simulink model "Acquisition_from_autosave"  (R2017a)
settings: Solver=VariableStepAuto  StartTime=0.0  StopTime=0.5  RelTol=1e-3
undefined symbols (not defined in the file): magnitude, Radix
libraries: simulink x34, commfilt2 x30, dspswit3 x12, dspmtrx3 x12, dspxfrm3 x3, simulink_extras x2, dspbuff3 x1
(part 3 of 4)

== system Acquisition_from_autosave/Tracking Loop/Tracking Loops/Tracking Loop3/Code Filter/Coeffiecients ==
  BW : Inport
  Zeta : Inport  Port=2
  ts : Inport  Port=3
  Constant1 : Constant  Value=2
  Divide1 : Product  Inputs=**/
  Math Function : Math  Operator=square  SaturateOnIntegerOverflow=on
  Math Function1 : Math  Operator=reciprocal  SaturateOnIntegerOverflow=on
  Wn : Subsystem
  "calc1 " : Subsystem
  calc2 : Product  Inputs=/*
  C1 : Outport
  C2 : Outport  Port=2
  wires:
  BW/1 -> Wn/1(BW)
  Zeta/1 -> Divide1/2, Wn/2(Zeta)
  Math Function/1 -> Math Function1/1
  Constant1/1 -> "calc1 "/1(2), Divide1/1
  Math Function1/1 -> "calc1 "/3(t1), calc2/1
  "calc1 "/1(Out1) -> C1/1
  calc2/1 -> C2/1
  Divide1/1 -> "calc1 "/2(t2)
  Wn/1(Wn) -> Divide1/3, Math Function/1
  ts/1 -> "calc1 "/4(ts), calc2/2

== system Acquisition_from_autosave/Tracking Loop/Tracking Loops/Tracking Loop3/PRN Generator /CA_Code  ==
  In1 : Inport
  CA_Code : MATLAB Function  TreatAsAtomicUnit=on  SystemSampleTime=0.001
  Constant1 : Constant  Value=32
  RT : RateTransition  OutPortSampleTime=0.001
  Reshape : Reshape  OutputDimensionality=Column vector (2-D)
  Out1 : Outport
  wires:
  In1/1 -> RT/1
  CA_Code/1(g) -> Reshape/1
  Constant1/1 -> CA_Code/2(fs)
  Reshape/1 -> Out1/1
  RT/1 -> CA_Code/1(sv)

== system Acquisition_from_autosave/Tracking Loop/Tracking Loops/Tracking Loop3/PRN Generator /NRZ ==
  In1 : Inport
  Constant5 : Constant  Value=2  SampleTime=-1
  Constant6 : Constant  Value=-1
  Product4 : Product
  Sum4 : Sum  Inputs=|++
  Out1 : Outport
  wires:
  Constant6/1 -> Sum4/1
  Sum4/1 -> Out1/1
  Product4/1 -> Sum4/2
  In1/1 -> Product4/2
  Constant5/1 -> Product4/1

== system Acquisition_from_autosave/Tracking Loop/Tracking Loops/Tracking Loop4/Carrier Filter/Filter Parameters ==
  BW : Constant  Value=25
  Constant : Constant  Value=8
  Constant1 : Constant  Value=4
  Constant2 : Constant
  Constant3 : Constant  Value=2
  Damping : Constant  Value=0.707
  Divide : Product  Inputs=*/
  Gain 1 : Product  Inputs=***/
  Gain 2 : Product  Inputs=**/
  K : Constant
  Product : Product  Inputs=3
  Product1 : Product  Inputs=3
  Sum : Sum  Inputs=|++
  K1 : Outport
  K2 : Outport  Port=2
  wires:
  Damping/1 -> Gain 1/3, Product1/2, Product1/1, Product/3
  K/1 -> Gain 2/3, Gain 1/4
  BW/1 -> Product/2
  Constant/1 -> Product/1
  Product/1 -> Divide/1
  Constant1/1 -> Product1/3
  Constant2/1 -> Sum/1
  Product1/1 -> Sum/2
  Sum/1 -> Divide/2
  Divide/1 -> Gain 2/2, Gain 2/1, Gain 1/1
  Constant3/1 -> Gain 1/2
  Gain 1/1 -> K1/1
  Gain 2/1 -> K2/1

== system Acquisition_from_autosave/Tracking Loop/Tracking Loops/Tracking Loop4/Carrier Filter/Subsystem ==
  BW : Constant  Value=30
  C1 : Subsystem
  C2 : Subsystem
  Constant1 : Constant  Value=8
  Constant2 : Constant  Value=4
  Constant4 : Constant
  Damping : Constant  Value=0.707
  K : Constant  Value=4
  T : Constant  Value=0.001
  Wn : Subsystem
  "K2 " : Outport
  K1 : Outport  Port=2
  wires:
  C1/1(Out1) -> K1/1
  Constant1/1 -> C1/1(In1), Wn/1(In1)
  BW/1 -> Wn/2(In2)
  Damping/1 -> C1/2(In2), C1/3(In3), Wn/3(In3), C2/3(In3), C2/2(In2)
  Constant2/1 -> C2/5(In5), C1/7(In7), C2/6(In6), C2/7(In7), C1/8(In8), Wn/4(In4)
  Constant4/1 -> Wn/5(In5)
  T/1 -> C1/4(In4), C1/5(In5), C1/6(In6), C2/4(In4)
  Wn/1(Out1) -> C1/10(In10), C2/8(In8), C1/9(In9)
  C2/1(Out1) -> "K2 "/1
  K/1 -> C1/11(In11), C2/1(In1)

== system Acquisition_from_autosave/Tracking Loop/Tracking Loops/Tracking Loop4/Code Filter/Coeffiecients ==
  BW : Inport
  Zeta : Inport  Port=2
  ts : Inport  Port=3
  Constant1 : Constant  Value=2
  Divide1 : Product  Inputs=**/
  Math Function : Math  Operator=square  SaturateOnIntegerOverflow=on
  Math Function1 : Math  Operator=reciprocal  SaturateOnIntegerOverflow=on
  Wn : Subsystem
  "calc1 " : Subsystem
  calc2 : Product  Inputs=/*
  C1 : Outport
  C2 : Outport  Port=2
  wires:
  BW/1 -> Wn/1(BW)
  Zeta/1 -> Divide1/2, Wn/2(Zeta)
  Math Function/1 -> Math Function1/1
  Constant1/1 -> "calc1 "/1(2), Divide1/1
  Math Function1/1 -> "calc1 "/3(t1), calc2/1
  "calc1 "/1(Out1) -> C1/1
  calc2/1 -> C2/1
  Divide1/1 -> "calc1 "/2(t2)
  Wn/1(Wn) -> Divide1/3, Math Function/1
  ts/1 -> "calc1 "/4(ts), calc2/2

== system Acquisition_from_autosave/Tracking Loop/Tracking Loops/Tracking Loop4/PRN Generator /CA_Code  ==
  In1 : Inport
  CA_Code : MATLAB Function  TreatAsAtomicUnit=on  SystemSampleTime=0.001
  Constant1 : Constant  Value=32
  RT : RateTransition  OutPortSampleTime=0.001
  Reshape : Reshape  OutputDimensionality=Column vector (2-D)
  Out1 : Outport
  wires:
  In1/1 -> RT/1
  CA_Code/1(g) -> Reshape/1
  Constant1/1 -> CA_Code/2(fs)
  Reshape/1 -> Out1/1
  RT/1 -> CA_Code/1(sv)

== system Acquisition_from_autosave/Tracking Loop/Tracking Loops/Tracking Loop4/PRN Generator /NRZ ==
  In1 : Inport
  Constant5 : Constant  Value=2  SampleTime=-1
  Constant6 : Constant  Value=-1
  Product4 : Product
  Sum4 : Sum  Inputs=|++
  Out1 : Outport
  wires:
  Constant6/1 -> Sum4/1
  Sum4/1 -> Out1/1
  Product4/1 -> Sum4/2
  In1/1 -> Product4/2
  Constant5/1 -> Product4/1

== system Acquisition_from_autosave/Tracking Loop/Tracking Loops/Tracking Loop5/Carrier Filter/Filter Parameters ==
  BW : Constant  Value=25
  Constant : Constant  Value=8
  Constant1 : Constant  Value=4
  Constant2 : Constant
  Constant3 : Constant  Value=2
  Damping : Constant  Value=0.707
  Divide : Product  Inputs=*/
  Gain 1 : Product  Inputs=***/
  Gain 2 : Product  Inputs=**/
  K : Constant
  Product : Product  Inputs=3
  Product1 : Product  Inputs=3
  Sum : Sum  Inputs=|++
  K1 : Outport
  K2 : Outport  Port=2
  wires:
  Damping/1 -> Gain 1/3, Product1/2, Product1/1, Product/3
  K/1 -> Gain 2/3, Gain 1/4
  BW/1 -> Product/2
  Constant/1 -> Product/1
  Product/1 -> Divide/1
  Constant1/1 -> Product1/3
  Constant2/1 -> Sum/1
  Product1/1 -> Sum/2
  Sum/1 -> Divide/2
  Divide/1 -> Gain 2/2, Gain 2/1, Gain 1/1
  Constant3/1 -> Gain 1/2
  Gain 1/1 -> K1/1
  Gain 2/1 -> K2/1

== system Acquisition_from_autosave/Tracking Loop/Tracking Loops/Tracking Loop5/Carrier Filter/Subsystem ==
  BW : Constant  Value=30
  C1 : Subsystem
  C2 : Subsystem
  Constant1 : Constant  Value=8
  Constant2 : Constant  Value=4
  Constant4 : Constant
  Damping : Constant  Value=0.707
  K : Constant  Value=4
  T : Constant  Value=0.001
  Wn : Subsystem
  "K2 " : Outport
  K1 : Outport  Port=2
  wires:
  C1/1(Out1) -> K1/1
  Constant1/1 -> C1/1(In1), Wn/1(In1)
  BW/1 -> Wn/2(In2)
  Damping/1 -> C1/2(In2), C1/3(In3), Wn/3(In3), C2/3(In3), C2/2(In2)
  Constant2/1 -> C2/5(In5), C1/7(In7), C2/6(In6), C2/7(In7), C1/8(In8), Wn/4(In4)
  Constant4/1 -> Wn/5(In5)
  T/1 -> C1/4(In4), C1/5(In5), C1/6(In6), C2/4(In4)
  Wn/1(Out1) -> C1/10(In10), C2/8(In8), C1/9(In9)
  C2/1(Out1) -> "K2 "/1
  K/1 -> C1/11(In11), C2/1(In1)

== system Acquisition_from_autosave/Tracking Loop/Tracking Loops/Tracking Loop5/Code Filter/Coeffiecients ==
  BW : Inport
  Zeta : Inport  Port=2
  ts : Inport  Port=3
  Constant1 : Constant  Value=2
  Divide1 : Product  Inputs=**/
  Math Function : Math  Operator=square  SaturateOnIntegerOverflow=on
  Math Function1 : Math  Operator=reciprocal  SaturateOnIntegerOverflow=on
  Wn : Subsystem
  "calc1 " : Subsystem
  calc2 : Product  Inputs=/*
  C1 : Outport
  C2 : Outport  Port=2
  wires:
  BW/1 -> Wn/1(BW)
  Zeta/1 -> Divide1/2, Wn/2(Zeta)
  Math Function/1 -> Math Function1/1
  Constant1/1 -> "calc1 "/1(2), Divide1/1
  Math Function1/1 -> "calc1 "/3(t1), calc2/1
  "calc1 "/1(Out1) -> C1/1
  calc2/1 -> C2/1
  Divide1/1 -> "calc1 "/2(t2)
  Wn/1(Wn) -> Divide1/3, Math Function/1
  ts/1 -> "calc1 "/4(ts), calc2/2

== system Acquisition_from_autosave/Tracking Loop/Tracking Loops/Tracking Loop5/PRN Generator /CA_Code  ==
  In1 : Inport
  CA_Code : MATLAB Function  TreatAsAtomicUnit=on  SystemSampleTime=0.001
  Constant1 : Constant  Value=32
  RT : RateTransition  OutPortSampleTime=0.001
  Reshape : Reshape  OutputDimensionality=Column vector (2-D)
  Out1 : Outport
  wires:
  In1/1 -> RT/1
  CA_Code/1(g) -> Reshape/1
  Constant1/1 -> CA_Code/2(fs)
  Reshape/1 -> Out1/1
  RT/1 -> CA_Code/1(sv)

== system Acquisition_from_autosave/Tracking Loop/Tracking Loops/Tracking Loop5/PRN Generator /NRZ ==
  In1 : Inport
  Constant5 : Constant  Value=2  SampleTime=-1
  Constant6 : Constant  Value=-1
  Product4 : Product
  Sum4 : Sum  Inputs=|++
  Out1 : Outport
  wires:
  Constant6/1 -> Sum4/1
  Sum4/1 -> Out1/1
  Product4/1 -> Sum4/2
  In1/1 -> Product4/2
  Constant5/1 -> Product4/1

== system Acquisition_from_autosave/Tracking Loop/Tracking Loops/Tracking Loop1/Carrier Filter/Subsystem/C1 ==
  In1 : Inport
  In2 : Inport  Port=2
  In3 : Inport  Port=3
  In4 : Inport  Port=4
  In5 : Inport  Port=5
  In6 : Inport  Port=6
  In7 : Inport  Port=7
  In8 : Inport  Port=8
  In9 : Inport  Port=9
  In10 : Inport  Port=10
  In11 : Inport  Port=11
  Add1 : Sum  Inputs=+++
  Gain 3 : Product  Inputs=***/
  Gain 4 : Product  Inputs=***
  Math Function3 : Math  Operator=square  SaturateOnIntegerOverflow=on
  Product3 : Product
  Product4 : Product  Inputs=4
  Out1 : Outport
  wires:
  In5/1 -> Product4/4
  In7/1 -> Add1/3
  Gain 3/1 -> Out1/1
  In9/1 -> Product4/3
  In4/1 -> Product3/1
  In8/1 -> Product4/1
  In2/1 -> Gain 4/1
  In11/1 -> Gain 3/1
  In10/1 -> Product3/2, Gain 4/2
  In1/1 -> Gain 3/3
  In6/1 -> Gain 4/3
  In3/1 -> Product4/2
  Add1/1 -> Gain 3/4
  Product4/1 -> Add1/2
  Gain 4/1 -> Gain 3/2
  Math Function3/1 -> Add1/1
  Product3/1 -> Math Function3/1

== system Acquisition_from_autosave/Tracking Loop/Tracking Loops/Tracking Loop1/Carrier Filter/Subsystem/C2 ==
  In1 : Inport
  In2 : Inport  Port=2
  In3 : Inport  Port=3
  In4 : Inport  Port=4
  In5 : Inport  Port=5
  In6 : Inport  Port=6
  In7 : Inport  Port=7
  In8 : Inport  Port=8
  Add : Sum  Inputs=+++
  Gain 1 : Product  Inputs=***/
  Gain 2 : Product  Inputs=***
  Math Function : Math  Operator=square  SaturateOnIntegerOverflow=on
  Math Function1 : Math  Operator=square  SaturateOnIntegerOverflow=on
  Product1 : Product
  Product2 : Product  Inputs=4
  Out1 : Outport
  wires:
  Product1/1 -> Math Function1/1
  Math Function1/1 -> Add/1
  Add/1 -> Gain 1/4
  In2/1 -> Gain 2/1
  In5/1 -> Add/3
  In7/1 -> Product2/1
  In3/1 -> Product2/2
  In1/1 -> Gain 1/3
  In6/1 -> Gain 1/2
  Product2/1 -> Add/2
  Gain 1/1 -> Out1/1
  Math Function/1 -> Gain 1/1
  In8/1 -> Product1/1, Gain 2/2, Product2/3
  In4/1 -> Product1/2, Product2/4, Gain 2/3
  Gain 2/1 -> Math Function/1

== system Acquisition_from_autosave/Tracking Loop/Tracking Loops/Tracking Loop1/Carrier Filter/Subsystem/Wn ==
  In1 : Inport
  In2 : Inport  Port=2
  In3 : Inport  Port=3
  In4 : Inport  Port=4
  In5 : Inport  Port=5
  Add : Sum
  Divide1 : Product  Inputs=***/
  Math Function : Math  Operator=square  SaturateOnIntegerOverflow=on
  Wn1 : Product
  Out1 : Outport
  wires:
  In4/1 -> Wn1/2
  Add/1 -> Divide1/4
  Wn1/1 -> Add/1
  In3/1 -> Divide1/3, Math Function/1
  In2/1 -> Divide1/2
  Math Function/1 -> Wn1/1
  Divide1/1 -> Out1/1
  In1/1 -> Divide1/1
  In5/1 -> Add/2

== system Acquisition_from_autosave/Tracking Loop/Tracking Loops/Tracking Loop1/Filter/Subsystem/C1 ==
  In1 : Inport
  In2 : Inport  Port=2
  In3 : Inport  Port=3
  In4 : Inport  Port=4
  In5 : Inport  Port=5
  In6 : Inport  Port=6
  In7 : Inport  Port=7
  In8 : Inport  Port=8
  In9 : Inport  Port=9
  In10 : Inport  Port=10
  In11 : Inport  Port=11
  Add1 : Sum  Inputs=+++
  Gain 3 : Product  Inputs=***/
  Gain 4 : Product  Inputs=***
  Math Function3 : Math  Operator=square  SaturateOnIntegerOverflow=on
  Product3 : Product
  Product4 : Product  Inputs=4
  Out1 : Outport
  wires:
  In5/1 -> Product4/4
  In7/1 -> Add1/3
  Gain 3/1 -> Out1/1
  In9/1 -> Product4/3
  In4/1 -> Product3/1
  In8/1 -> Product4/1
  In2/1 -> Gain 4/1
  In11/1 -> Gain 3/1
  In10/1 -> Product3/2, Gain 4/2
  In1/1 -> Gain 3/3
  In6/1 -> Gain 4/3
  In3/1 -> Product4/2
  Add1/1 -> Gain 3/4
  Product4/1 -> Add1/2
  Gain 4/1 -> Gain 3/2
  Math Function3/1 -> Add1/1
  Product3/1 -> Math Function3/1

== system Acquisition_from_autosave/Tracking Loop/Tracking Loops/Tracking Loop1/Filter/Subsystem/C2 ==
  In1 : Inport
  In2 : Inport  Port=2
  In3 : Inport  Port=3
  In4 : Inport  Port=4
  In5 : Inport  Port=5
  In6 : Inport  Port=6
  In7 : Inport  Port=7
  In8 : Inport  Port=8
  Add : Sum  Inputs=+++
  Gain 1 : Product  Inputs=***/
  Gain 2 : Product  Inputs=***
  Math Function : Math  Operator=square  SaturateOnIntegerOverflow=on
  Math Function1 : Math  Operator=square  SaturateOnIntegerOverflow=on
  Product1 : Product
  Product2 : Product  Inputs=4
  Out1 : Outport
  wires:
  Product1/1 -> Math Function1/1
  Math Function1/1 -> Add/1
  Add/1 -> Gain 1/4
  In2/1 -> Gain 2/1
  In5/1 -> Add/3
  In7/1 -> Product2/1
  In3/1 -> Product2/2
  In1/1 -> Gain 1/3
  In6/1 -> Gain 1/2
  Product2/1 -> Add/2
  Gain 1/1 -> Out1/1
  Math Function/1 -> Gain 1/1
  In8/1 -> Product1/1, Gain 2/2, Product2/3
  In4/1 -> Product1/2, Product2/4, Gain 2/3
  Gain 2/1 -> Math Function/1

== system Acquisition_from_autosave/Tracking Loop/Tracking Loops/Tracking Loop1/Filter/Subsystem/Wn ==
  In1 : Inport
  In2 : Inport  Port=2
  In3 : Inport  Port=3
  In4 : Inport  Port=4
  In5 : Inport  Port=5
  Add : Sum
  Divide1 : Product  Inputs=***/
  Math Function : Math  Operator=square  SaturateOnIntegerOverflow=on
  Wn1 : Product
  Out1 : Outport
  wires:
  In4/1 -> Wn1/2
  Add/1 -> Divide1/4
  Wn1/1 -> Add/1
  In3/1 -> Divide1/3, Math Function/1
  In2/1 -> Divide1/2
  Math Function/1 -> Wn1/1
  Divide1/1 -> Out1/1
  In1/1 -> Divide1/1
  In5/1 -> Add/2

== system Acquisition_from_autosave/Tracking Loop/Tracking Loops/Tracking Loop2/Carrier Filter/Subsystem/C1 ==
  In1 : Inport
  In2 : Inport  Port=2
  In3 : Inport  Port=3
  In4 : Inport  Port=4
  In5 : Inport  Port=5
  In6 : Inport  Port=6
  In7 : Inport  Port=7
  In8 : Inport  Port=8
  In9 : Inport  Port=9
  In10 : Inport  Port=10
  In11 : Inport  Port=11
  Add1 : Sum  Inputs=+++
  Gain 3 : Product  Inputs=***/
  Gain 4 : Product  Inputs=***
  Math Function3 : Math  Operator=square  SaturateOnIntegerOverflow=on
  Product3 : Product
  Product4 : Product  Inputs=4
  Out1 : Outport
  wires:
  In5/1 -> Product4/4
  In7/1 -> Add1/3
  Gain 3/1 -> Out1/1
  In9/1 -> Product4/3
  In4/1 -> Product3/1
  In8/1 -> Product4/1
  In2/1 -> Gain 4/1
  In11/1 -> Gain 3/1
  In10/1 -> Product3/2, Gain 4/2
  In1/1 -> Gain 3/3
  In6/1 -> Gain 4/3
  In3/1 -> Product4/2
  Add1/1 -> Gain 3/4
  Product4/1 -> Add1/2
  Gain 4/1 -> Gain 3/2
  Math Function3/1 -> Add1/1
  Product3/1 -> Math Function3/1

== system Acquisition_from_autosave/Tracking Loop/Tracking Loops/Tracking Loop2/Carrier Filter/Subsystem/C2 ==
  In1 : Inport
  In2 : Inport  Port=2
  In3 : Inport  Port=3
  In4 : Inport  Port=4
  In5 : Inport  Port=5
  In6 : Inport  Port=6
  In7 : Inport  Port=7
  In8 : Inport  Port=8
  Add : Sum  Inputs=+++
  Gain 1 : Product  Inputs=***/
  Gain 2 : Product  Inputs=***
  Math Function : Math  Operator=square  SaturateOnIntegerOverflow=on
  Math Function1 : Math  Operator=square  SaturateOnIntegerOverflow=on
  Product1 : Product
  Product2 : Product  Inputs=4
  Out1 : Outport
  wires:
  Product1/1 -> Math Function1/1
  Math Function1/1 -> Add/1
  Add/1 -> Gain 1/4
  In2/1 -> Gain 2/1
  In5/1 -> Add/3
  In7/1 -> Product2/1
  In3/1 -> Product2/2
  In1/1 -> Gain 1/3
  In6/1 -> Gain 1/2
  Product2/1 -> Add/2
  Gain 1/1 -> Out1/1
  Math Function/1 -> Gain 1/1
  In8/1 -> Product1/1, Gain 2/2, Product2/3
  In4/1 -> Product1/2, Product2/4, Gain 2/3
  Gain 2/1 -> Math Function/1

== system Acquisition_from_autosave/Tracking Loop/Tracking Loops/Tracking Loop2/Carrier Filter/Subsystem/Wn ==
  In1 : Inport
  In2 : Inport  Port=2
  In3 : Inport  Port=3
  In4 : Inport  Port=4
  In5 : Inport  Port=5
  Add : Sum
  Divide1 : Product  Inputs=***/
  Math Function : Math  Operator=square  SaturateOnIntegerOverflow=on
  Wn1 : Product
  Out1 : Outport
  wires:
  In4/1 -> Wn1/2
  Add/1 -> Divide1/4
  Wn1/1 -> Add/1
  In3/1 -> Divide1/3, Math Function/1
  In2/1 -> Divide1/2
  Math Function/1 -> Wn1/1
  Divide1/1 -> Out1/1
  In1/1 -> Divide1/1
  In5/1 -> Add/2

== system Acquisition_from_autosave/Tracking Loop/Tracking Loops/Tracking Loop2/Code Filter/Coeffiecients/Wn ==
  BW : Inport
  Zeta : Inport  Port=2
  Constant1 : Constant  Value=8
  Constant2 : Constant  Value=4
  Constant3 : Constant
  Divide1 : Product  Inputs=*/
  Math Function : Math  Operator=square  SaturateOnIntegerOverflow=on
  Product : Product
  Product1 : Product  Inputs=3
  Sum3 : Sum  Inputs=|++
  Wn : Outport
  wires:
  Constant2/1 -> Product/2
  Divide1/1 -> Wn/1
  Product1/1 -> Divide1/1
  Math Function/1 -> Product/1
  Product/1 -> Sum3/1
  BW/1 -> Product1/1
  Sum3/1 -> Divide1/2
  Constant3/1 -> Sum3/2
  Zeta/1 -> Product1/3, Math Function/1
  Constant1/1 -> Product1/2

== system Acquisition_from_autosave/Tracking Loop/Tracking Loops/Tracking Loop2/Code Filter/Coeffiecients/calc1  ==
  2 : Inport
  t2 : Inport  Port=2
  t1 : Inport  Port=3
  ts : Inport  Port=4
  Divide3 : Product  Inputs=**
  Divide4 : Product  Inputs=**
  Divide5 : Product  Inputs=/*
  Subtract : Sum  Inputs=+-
  Out1 : Outport
  wires:
  2/1 -> Divide4/1, Divide3/1
  ts/1 -> Subtract/2
  t1/1 -> Divide4/2
  Divide5/1 -> Out1/1
  Subtract/1 -> Divide5/2
  Divide4/1 -> Divide5/1
  t2/1 -> Divide3/2
  Divide3/1 -> Subtract/1

== system Acquisition_from_autosave/Tracking Loop/Tracking Loops/Tracking Loop3/Carrier Filter/Subsystem/C1 ==
  In1 : Inport
  In2 : Inport  Port=2
  In3 : Inport  Port=3
  In4 : Inport  Port=4
  In5 : Inport  Port=5
  In6 : Inport  Port=6
  In7 : Inport  Port=7
  In8 : Inport  Port=8
  In9 : Inport  Port=9
  In10 : Inport  Port=10
  In11 : Inport  Port=11
  Add1 : Sum  Inputs=+++
  Gain 3 : Product  Inputs=***/
  Gain 4 : Product  Inputs=***
  Math Function3 : Math  Operator=square  SaturateOnIntegerOverflow=on
  Product3 : Product
  Product4 : Product  Inputs=4
  Out1 : Outport
  wires:
  In5/1 -> Product4/4
  In7/1 -> Add1/3
  Gain 3/1 -> Out1/1
  In9/1 -> Product4/3
  In4/1 -> Product3/1
  In8/1 -> Product4/1
  In2/1 -> Gain 4/1
  In11/1 -> Gain 3/1
  In10/1 -> Product3/2, Gain 4/2
  In1/1 -> Gain 3/3
  In6/1 -> Gain 4/3
  In3/1 -> Product4/2
  Add1/1 -> Gain 3/4
  Product4/1 -> Add1/2
  Gain 4/1 -> Gain 3/2
  Math Function3/1 -> Add1/1
  Product3/1 -> Math Function3/1

== system Acquisition_from_autosave/Tracking Loop/Tracking Loops/Tracking Loop3/Carrier Filter/Subsystem/C2 ==
  In1 : Inport
  In2 : Inport  Port=2
  In3 : Inport  Port=3
  In4 : Inport  Port=4
  In5 : Inport  Port=5
  In6 : Inport  Port=6
  In7 : Inport  Port=7
  In8 : Inport  Port=8
  Add : Sum  Inputs=+++
  Gain 1 : Product  Inputs=***/
  Gain 2 : Product  Inputs=***
  Math Function : Math  Operator=square  SaturateOnIntegerOverflow=on
  Math Function1 : Math  Operator=square  SaturateOnIntegerOverflow=on
  Product1 : Product
  Product2 : Product  Inputs=4
  Out1 : Outport
  wires:
  Product1/1 -> Math Function1/1
  Math Function1/1 -> Add/1
  Add/1 -> Gain 1/4
  In2/1 -> Gain 2/1
  In5/1 -> Add/3
  In7/1 -> Product2/1
  In3/1 -> Product2/2
  In1/1 -> Gain 1/3
  In6/1 -> Gain 1/2
  Product2/1 -> Add/2
  Gain 1/1 -> Out1/1
  Math Function/1 -> Gain 1/1
  In8/1 -> Product1/1, Gain 2/2, Product2/3
  In4/1 -> Product1/2, Product2/4, Gain 2/3
  Gain 2/1 -> Math Function/1

== system Acquisition_from_autosave/Tracking Loop/Tracking Loops/Tracking Loop3/Carrier Filter/Subsystem/Wn ==
  In1 : Inport
  In2 : Inport  Port=2
  In3 : Inport  Port=3
  In4 : Inport  Port=4
  In5 : Inport  Port=5
  Add : Sum
  Divide1 : Product  Inputs=***/
  Math Function : Math  Operator=square  SaturateOnIntegerOverflow=on
  Wn1 : Product
  Out1 : Outport
  wires:
  In4/1 -> Wn1/2
  Add/1 -> Divide1/4
  Wn1/1 -> Add/1
  In3/1 -> Divide1/3, Math Function/1
  In2/1 -> Divide1/2
  Math Function/1 -> Wn1/1
  Divide1/1 -> Out1/1
  In1/1 -> Divide1/1
  In5/1 -> Add/2

== system Acquisition_from_autosave/Tracking Loop/Tracking Loops/Tracking Loop3/Code Filter/Coeffiecients/Wn ==
  BW : Inport
  Zeta : Inport  Port=2
  Constant1 : Constant  Value=8
  Constant2 : Constant  Value=4
  Constant3 : Constant
  Divide1 : Product  Inputs=*/
  Math Function : Math  Operator=square  SaturateOnIntegerOverflow=on
  Product : Product
  Product1 : Product  Inputs=3
  Sum3 : Sum  Inputs=|++
  Wn : Outport
  wires:
  Constant2/1 -> Product/2
  Divide1/1 -> Wn/1
  Product1/1 -> Divide1/1
  Math Function/1 -> Product/1
  Product/1 -> Sum3/1
  BW/1 -> Product1/1
  Sum3/1 -> Divide1/2
  Constant3/1 -> Sum3/2
  Zeta/1 -> Product1/3, Math Function/1
  Constant1/1 -> Product1/2

== system Acquisition_from_autosave/Tracking Loop/Tracking Loops/Tracking Loop3/Code Filter/Coeffiecients/calc1  ==
  2 : Inport
  t2 : Inport  Port=2
  t1 : Inport  Port=3
  ts : Inport  Port=4
  Divide3 : Product  Inputs=**
  Divide4 : Product  Inputs=**
  Divide5 : Product  Inputs=/*
  Subtract : Sum  Inputs=+-
  Out1 : Outport
  wires:
  2/1 -> Divide4/1, Divide3/1
  ts/1 -> Subtract/2
  t1/1 -> Divide4/2
  Divide5/1 -> Out1/1
  Subtract/1 -> Divide5/2
  Divide4/1 -> Divide5/1
  t2/1 -> Divide3/2
  Divide3/1 -> Subtract/1

== system Acquisition_from_autosave/Tracking Loop/Tracking Loops/Tracking Loop4/Carrier Filter/Subsystem/C1 ==
  In1 : Inport
  In2 : Inport  Port=2
  In3 : Inport  Port=3
  In4 : Inport  Port=4
  In5 : Inport  Port=5
  In6 : Inport  Port=6
  In7 : Inport  Port=7
  In8 : Inport  Port=8
  In9 : Inport  Port=9
  In10 : Inport  Port=10
  In11 : Inport  Port=11
  Add1 : Sum  Inputs=+++
  Gain 3 : Product  Inputs=***/
  Gain 4 : Product  Inputs=***
  Math Function3 : Math  Operator=square  SaturateOnIntegerOverflow=on
  Product3 : Product
  Product4 : Product  Inputs=4
  Out1 : Outport
  wires:
  In5/1 -> Product4/4
  In7/1 -> Add1/3
  Gain 3/1 -> Out1/1
  In9/1 -> Product4/3
  In4/1 -> Product3/1
  In8/1 -> Product4/1
  In2/1 -> Gain 4/1
  In11/1 -> Gain 3/1
  In10/1 -> Product3/2, Gain 4/2
  In1/1 -> Gain 3/3
  In6/1 -> Gain 4/3
  In3/1 -> Product4/2
  Add1/1 -> Gain 3/4
  Product4/1 -> Add1/2
  Gain 4/1 -> Gain 3/2
  Math Function3/1 -> Add1/1
  Product3/1 -> Math Function3/1

== system Acquisition_from_autosave/Tracking Loop/Tracking Loops/Tracking Loop4/Carrier Filter/Subsystem/C2 ==
  In1 : Inport
  In2 : Inport  Port=2
  In3 : Inport  Port=3
  In4 : Inport  Port=4
  In5 : Inport  Port=5
  In6 : Inport  Port=6
  In7 : Inport  Port=7
  In8 : Inport  Port=8
  Add : Sum  Inputs=+++
  Gain 1 : Product  Inputs=***/
  Gain 2 : Product  Inputs=***
  Math Function : Math  Operator=square  SaturateOnIntegerOverflow=on
  Math Function1 : Math  Operator=square  SaturateOnIntegerOverflow=on
  Product1 : Product
  Product2 : Product  Inputs=4
  Out1 : Outport
  wires:
  Product1/1 -> Math Function1/1
  Math Function1/1 -> Add/1
  Add/1 -> Gain 1/4
  In2/1 -> Gain 2/1
  In5/1 -> Add/3
  In7/1 -> Product2/1
  In3/1 -> Product2/2
  In1/1 -> Gain 1/3
  In6/1 -> Gain 1/2
  Product2/1 -> Add/2
  Gain 1/1 -> Out1/1
  Math Function/1 -> Gain 1/1
  In8/1 -> Product1/1, Gain 2/2, Product2/3
  In4/1 -> Product1/2, Product2/4, Gain 2/3
  Gain 2/1 -> Math Function/1

== system Acquisition_from_autosave/Tracking Loop/Tracking Loops/Tracking Loop4/Carrier Filter/Subsystem/Wn ==
  In1 : Inport
  In2 : Inport  Port=2
  In3 : Inport  Port=3
  In4 : Inport  Port=4
  In5 : Inport  Port=5
  Add : Sum
  Divide1 : Product  Inputs=***/
  Math Function : Math  Operator=square  SaturateOnIntegerOverflow=on
  Wn1 : Product
  Out1 : Outport
  wires:
  In4/1 -> Wn1/2
  Add/1 -> Divide1/4
  Wn1/1 -> Add/1
  In3/1 -> Divide1/3, Math Function/1
  In2/1 -> Divide1/2
  Math Function/1 -> Wn1/1
  Divide1/1 -> Out1/1
  In1/1 -> Divide1/1
  In5/1 -> Add/2

== system Acquisition_from_autosave/Tracking Loop/Tracking Loops/Tracking Loop4/Code Filter/Coeffiecients/Wn ==
  BW : Inport
  Zeta : Inport  Port=2
  Constant1 : Constant  Value=8
  Constant2 : Constant  Value=4
  Constant3 : Constant
  Divide1 : Product  Inputs=*/
  Math Function : Math  Operator=square  SaturateOnIntegerOverflow=on
  Product : Product
  Product1 : Product  Inputs=3
  Sum3 : Sum  Inputs=|++
  Wn : Outport
  wires:
  Constant2/1 -> Product/2
  Divide1/1 -> Wn/1
  Product1/1 -> Divide1/1
  Math Function/1 -> Product/1
  Product/1 -> Sum3/1
  BW/1 -> Product1/1
  Sum3/1 -> Divide1/2
  Constant3/1 -> Sum3/2
  Zeta/1 -> Product1/3, Math Function/1
  Constant1/1 -> Product1/2

== system Acquisition_from_autosave/Tracking Loop/Tracking Loops/Tracking Loop4/Code Filter/Coeffiecients/calc1  ==
  2 : Inport
  t2 : Inport  Port=2
  t1 : Inport  Port=3
  ts : Inport  Port=4
  Divide3 : Product  Inputs=**
  Divide4 : Product  Inputs=**
  Divide5 : Product  Inputs=/*
  Subtract : Sum  Inputs=+-
  Out1 : Outport
  wires:
  2/1 -> Divide4/1, Divide3/1
  ts/1 -> Subtract/2
  t1/1 -> Divide4/2
  Divide5/1 -> Out1/1
  Subtract/1 -> Divide5/2
  Divide4/1 -> Divide5/1
  t2/1 -> Divide3/2
  Divide3/1 -> Subtract/1

== system Acquisition_from_autosave/Tracking Loop/Tracking Loops/Tracking Loop5/Carrier Filter/Subsystem/C1 ==
  In1 : Inport
  In2 : Inport  Port=2
  In3 : Inport  Port=3
  In4 : Inport  Port=4
  In5 : Inport  Port=5
  In6 : Inport  Port=6
  In7 : Inport  Port=7
  In8 : Inport  Port=8
  In9 : Inport  Port=9
  In10 : Inport  Port=10
  In11 : Inport  Port=11
  Add1 : Sum  Inputs=+++
  Gain 3 : Product  Inputs=***/
  Gain 4 : Product  Inputs=***
  Math Function3 : Math  Operator=square  SaturateOnIntegerOverflow=on
  Product3 : Product
  Product4 : Product  Inputs=4
  Out1 : Outport
  wires:
  In5/1 -> Product4/4
  In7/1 -> Add1/3
  Gain 3/1 -> Out1/1
  In9/1 -> Product4/3
  In4/1 -> Product3/1
  In8/1 -> Product4/1
  In2/1 -> Gain 4/1
  In11/1 -> Gain 3/1
  In10/1 -> Product3/2, Gain 4/2
  In1/1 -> Gain 3/3
  In6/1 -> Gain 4/3
  In3/1 -> Product4/2
  Add1/1 -> Gain 3/4
  Product4/1 -> Add1/2
  Gain 4/1 -> Gain 3/2
  Math Function3/1 -> Add1/1
  Product3/1 -> Math Function3/1

== system Acquisition_from_autosave/Tracking Loop/Tracking Loops/Tracking Loop5/Carrier Filter/Subsystem/C2 ==
  In1 : Inport
  In2 : Inport  Port=2
  In3 : Inport  Port=3
  In4 : Inport  Port=4
  In5 : Inport  Port=5
  In6 : Inport  Port=6
  In7 : Inport  Port=7
  In8 : Inport  Port=8
  Add : Sum  Inputs=+++
  Gain 1 : Product  Inputs=***/
  Gain 2 : Product  Inputs=***
  Math Function : Math  Operator=square  SaturateOnIntegerOverflow=on
  Math Function1 : Math  Operator=square  SaturateOnIntegerOverflow=on
  Product1 : Product
  Product2 : Product  Inputs=4
  Out1 : Outport
  wires:
  Product1/1 -> Math Function1/1
  Math Function1/1 -> Add/1
  Add/1 -> Gain 1/4
  In2/1 -> Gain 2/1
  In5/1 -> Add/3
  In7/1 -> Product2/1
  In3/1 -> Product2/2
  In1/1 -> Gain 1/3
  In6/1 -> Gain 1/2
  Product2/1 -> Add/2
  Gain 1/1 -> Out1/1
  Math Function/1 -> Gain 1/1
  In8/1 -> Product1/1, Gain 2/2, Product2/3
  In4/1 -> Product1/2, Product2/4, Gain 2/3
  Gain 2/1 -> Math Function/1

== system Acquisition_from_autosave/Tracking Loop/Tracking Loops/Tracking Loop5/Carrier Filter/Subsystem/Wn ==
  In1 : Inport
  In2 : Inport  Port=2
  In3 : Inport  Port=3
  In4 : Inport  Port=4
  In5 : Inport  Port=5
  Add : Sum
  Divide1 : Product  Inputs=***/
  Math Function : Math  Operator=square  SaturateOnIntegerOverflow=on
  Wn1 : Product
  Out1 : Outport
  wires:
  In4/1 -> Wn1/2
  Add/1 -> Divide1/4
  Wn1/1 -> Add/1
  In3/1 -> Divide1/3, Math Function/1
  In2/1 -> Divide1/2
  Math Function/1 -> Wn1/1
  Divide1/1 -> Out1/1
  In1/1 -> Divide1/1
  In5/1 -> Add/2

== system Acquisition_from_autosave/Tracking Loop/Tracking Loops/Tracking Loop5/Code Filter/Coeffiecients/Wn ==
  BW : Inport
  Zeta : Inport  Port=2
  Constant1 : Constant  Value=8
  Constant2 : Constant  Value=4
  Constant3 : Constant
  Divide1 : Product  Inputs=*/
  Math Function : Math  Operator=square  SaturateOnIntegerOverflow=on
  Product : Product
  Product1 : Product  Inputs=3
  Sum3 : Sum  Inputs=|++
  Wn : Outport
  wires:
  Constant2/1 -> Product/2
  Divide1/1 -> Wn/1
  Product1/1 -> Divide1/1
  Math Function/1 -> Product/1
  Product/1 -> Sum3/1
  BW/1 -> Product1/1
  Sum3/1 -> Divide1/2
  Constant3/1 -> Sum3/2
  Zeta/1 -> Product1/3, Math Function/1
  Constant1/1 -> Product1/2

== system Acquisition_from_autosave/Tracking Loop/Tracking Loops/Tracking Loop5/Code Filter/Coeffiecients/calc1  ==
  2 : Inport
  t2 : Inport  Port=2
  t1 : Inport  Port=3
  ts : Inport  Port=4
  Divide3 : Product  Inputs=**
  Divide4 : Product  Inputs=**
  Divide5 : Product  Inputs=/*
  Subtract : Sum  Inputs=+-
  Out1 : Outport
  wires:
  2/1 -> Divide4/1, Divide3/1
  ts/1 -> Subtract/2
  t1/1 -> Divide4/2
  Divide5/1 -> Out1/1
  Subtract/1 -> Divide5/2
  Divide4/1 -> Divide5/1
  t2/1 -> Divide3/2
  Divide3/1 -> Subtract/1

== matlab function Acquisition_from_autosave/Acquisition/Array of Sattelite Info ==
  data: input_vector input; Visible_Satellites output; Complete output
function [Visible_Satellites, Complete]= sort_store(input_vector)
persistent output_vector;
persistent found;
persistent find4;
threshold = 2*10^7;
if isempty(find4)
    find4=0;
end
if isempty(found)
    found=0;
end
if isempty(output_vector)
    output_vector=zeros(6,4);
end

if input_vector(1,1)>threshold
    for x = 1:6
        if output_vector(x,1)== 0
    output_vector(x,1)=input_vector(1,1); %Correlation Value
    output_vector(x,2)=input_vector(2,1); %PRN
    output_vector(x,3)=input_vector(3,1); %Frequency
    output_vector(x,4)=input_vector(4,1); %Code Phase
    found=found+1;
         break
        end
    end
end
if (found>=4)
    find4=1;
end
Complete=find4;
Visible_Satellites = output_vector;

== matlab function Acquisition_from_autosave/Acquisition/Search Correlation Data/MATLAB Function ==
  data: vector input; Sat output; PRN input; freq_step input
function Sat = find(vector, PRN, freq_step)
PRN=PRN+1;
freq_step=freq_step-1;
Freq =9207000+freq_step*500-5000;
persistent PRN_prev;
if isempty(PRN_prev)
    PRN_prev=0;
end
persistent sat_vector;
if isempty(sat_vector)
    sat_vector=zeros(5,1);
end
if PRN_prev ~= PRN
    sat_vector(1,1)=0;
    sat_vector(2,1)=0;
    sat_vector(3,1)=0;
    sat_vector(4,1)=0;
    sat_vector(5,1)=0;
end
for x = 1:32768
    if (vector(x,1) >= sat_vector(1,1))
       sat_vector(1,1)=vector(x,1);
       sat_vector(2,1)=PRN;
       sat_vector(3,1)=Freq;    
       sat_vector(4,1)=floor((x-1)/32);
       sat_vector(5,1)=(freq_step);
    end
end 
PRN_prev=PRN;
Sat = sat_vector;

== matlab function Acquisition_from_autosave/Tracking Loop/Tracking Loops/Tracking Loop3/Controlled Carrier Generator/MATLAB Function ==
  data: time input; wave output; freq input; phase input
function wave = NCOGen(time, freq, phase)

wave = exp(1i*(2*pi*freq*time-mod(phase,2*pi)));

== matlab function Acquisition_from_autosave/Tracking Loop/Tracking Loops/Tracking Loop3/Controlled Carrier Generator/MATLAB Function1 ==
  data: f input; wave output; timer input; phase_error input
function wave = NCO(f, timer, phase_error)
wave = exp(1i*(2*pi*f*(timer+phase_error)));

== matlab function Acquisition_from_autosave/Tracking Loop/Tracking Loops/Tracking Loop3/Oscillator/MATLAB Function2 ==
  data: u input; I output; Q output
function [I,Q]= fcn(u)

I = cos(u);
Q = sin(u);

== matlab function Acquisition_from_autosave/Tracking Loop/Tracking Loops/Tracking Loop4/Controlled Carrier Generator/MATLAB Function ==
  data: time input; wave output; freq input; phase input
function wave = NCOGen(time, freq, phase)

wave = exp(1i*(2*pi*freq*time-mod(phase,2*pi)));

== matlab function Acquisition_from_autosave/Tracking Loop/Tracking Loops/Tracking Loop2/Controlled Carrier Generator/MATLAB Function ==
  data: time input; wave output; freq input; phase input
function wave = NCOGen(time, freq, phase)

wave = exp(1i*(2*pi*freq*time-mod(phase,2*pi)));

== matlab function Acquisition_from_autosave/Tracking Loop/Tracking Loops/Tracking Loop2/Controlled Carrier Generator/MATLAB Function1 ==
  data: f input; wave output; timer input; phase_error input
function wave = NCO(f, timer, phase_error)
wave = exp(1i*(2*pi*f*(timer+phase_error)));

== matlab function Acquisition_from_autosave/Tracking Loop/Tracking Loops/Tracking Loop2/Oscillator/MATLAB Function2 ==
  data: u input; I output; Q output
function [I,Q]= fcn(u)

I = cos(u);
Q = sin(u);

== matlab function Acquisition_from_autosave/Tracking Loop/Tracking Loops/Tracking Loop2/PRN Generator /CA_Code /CA_Code ==
  data: sv input; g output; fs input
function g=CAcode(sv,fs)
coder.extrinsic('warning')
% function G=CACODE(SV,FS) 
% Generates 1023 length C/A Codes for GPS PRNs 1-37
%
% 
% g: nx1023 matrix- with each PRN in each row with symbols 1 and 0
% sv: a row or column vector of the SV's to be generated
% 	 valid entries are 1 to 37
% fs: optional number of samples per chip (defaults to 1), fractional samples allowed, must be 1 or greater.
%
% For multiple samples per chip, function is a zero order hold. 
%
%
% For example to generate the C/A codes for PRN 6 and PRN 12 use:
% g=cacode([6 12]),
% and to generate the C/A codes for PRN 6 and PRN 12 at 5 MHz use
% g=cacode([6 12],5/1.023)
% 
%
% For more information refer to the "GPS SPS Signal Specification"
% http://www.navcen.uscg.gov/pubs/gps/sigspec/default.htm
%
% Dan Boschen 12-30-2007
% boschen@loglin.com

% Revision History
% rev 1.0 Dan Boschen 4-15-2007  Initial Release
%
% rev 1.1 Dan Boschen 7-15-2007  Corrected error with taps for PRN30, should be [2,7] was 
% 					incorrect as [1 7]. Thank you Jadah Zak for finding this.
%
%
% rev 1.2 Dan Boschen 12-26-2007 Fixed column index error when ceil ~ L 
%				Thank you Jared Meadows for finding this.
%
% rev 1.3 Dan Boschen 12-30-2007 Changed comment "first order hold" to
% "zero order hold".
%
% rev 1.4 Dan Boschen 6-1-2010   Updated email address in comments



if nargin<2
	fs=1;
end


if (max(sv)>37) || (min(sv)<1) || (min(size(sv))~=1)
	error('sv must be a row or column vector with integers between 1 and 37\n')
end

if fs<1
	error('fs must be 1 or greater\n')
end	

% force integers
testint=round(sv)-sv;
if testint ~= 0 
	warning('non-integer value entered for sv, rounding to closest integer\n');
	sv = round(sv);
end


% table of C/A Code Tap Selection (sets delay for G2 generator)
tap=[2 6;
    3 7;
    4 8;
    5 9;
    1 9;
    2 10;
    1 8;
    2 9;
    3 10;
    2 3;
    3 4;
    5 6;
    6 7;
    7 8;
    8 9;
    9 10;
    1 4;
    2 5;
    3 6;
    4 7;
    5 8;
    6 9;
    1 3;
    4 6;
    5 7;
    6 8;
    7 9;
    8 10;
    1 6;
    2 7;
    3 8;
    4 9
    5 10
    4 10
    1 7
    2 8
    4 10];

% G1 LFSR: x^10+x^3+1
s=[0 0 1 0 0 0 0 0 0 1];
n=length(s);
g1=ones(1,n);	%initialization vector for G1

%g=ones(1,38192);
%g2=ones(1,38192);
%gfs=ones(1,38192);

g=ones(1,65536/2);
g2=ones(1,65536/2);
gfs=ones(1,65536/2);

L=2^n-1;

% G2j LFSR: x^10+x^9+x^8+x^6+x^3+x^2+1
t=[0 1 1 0 0 1 0 1 1 1];
q=ones(1,n);	%initialization vector for G2

% generate C/A Code sequences:
tap_sel=tap(sv,:);
for inc=1:L
    g2(:,inc)=mod(sum(q(tap_sel),2),2);
    g(:,inc)=mod(g1(n)+g2(:,inc),2);
   g1=[mod(sum(g1.*s),2) g1(1:n-1)];
   q=[mod(sum(q.*t),2) q(1:n-1)];
end

%upsample to desired rate
if fs~=1
	%fractional upsampling with zero order hold
	index=0;
	for cnt = 1/fs:1/fs:L
		index=index+1;
		if ceil(cnt) > L   %traps a floating point error in index
			gfs(:,index)=g(:,L);
		else
			gfs(:,index)=g(:,ceil(cnt));
		end
	end 
	g=gfs;
end

== matlab function Acquisition_from_autosave/Tracking Loop/Tracking Loops/Tracking Loop3/PRN Generator /CA_Code /CA_Code ==
  data: sv input; g output; fs input
function g=CAcode(sv,fs)
coder.extrinsic('warning')
% function G=CACODE(SV,FS) 
% Generates 1023 length C/A Codes for GPS PRNs 1-37
%
% 
% g: nx1023 matrix- with each PRN in each row with symbols 1 and 0
% sv: a row or column vector of the SV's to be generated
% 	 valid entries are 1 to 37
% fs: optional number of samples per chip (defaults to 1), fractional samples allowed, must be 1 or greater.
%
% For multiple samples per chip, function is a zero order hold. 
%
%
% For example to generate the C/A codes for PRN 6 and PRN 12 use:
% g=cacode([6 12]),
% and to generate the C/A codes for PRN 6 and PRN 12 at 5 MHz use
% g=cacode([6 12],5/1.023)
% 
%
% For more information refer to the "GPS SPS Signal Specification"
% http://www.navcen.uscg.gov/pubs/gps/sigspec/default.htm
%
% Dan Boschen 12-30-2007
% boschen@loglin.com

% Revision History
% rev 1.0 Dan Boschen 4-15-2007  Initial Release
%
% rev 1.1 Dan Boschen 7-15-2007  Corrected error with taps for PRN30, should be [2,7] was 
% 					incorrect as [1 7]. Thank you Jadah Zak for finding this.
%
%
% rev 1.2 Dan Boschen 12-26-2007 Fixed column index error when ceil ~ L 
%				Thank you Jared Meadows for finding this.
%
% rev 1.3 Dan Boschen 12-30-2007 Changed comment "first order hold" to
% "zero order hold".
%
% rev 1.4 Dan Boschen 6-1-2010   Updated email address in comments



if nargin<2
	fs=1;
end


if (max(sv)>37) || (min(sv)<1) || (min(size(sv))~=1)
	error('sv must be a row or column vector with integers between 1 and 37\n')
end

if fs<1
	error('fs must be 1 or greater\n')
end	

% force integers
testint=round(sv)-sv;
if testint ~= 0 
	warning('non-integer value entered for sv, rounding to closest integer\n');
	sv = round(sv);
end


% table of C/A Code Tap Selection (sets delay for G2 generator)
tap=[2 6;
    3 7;
    4 8;
    5 9;
    1 9;
    2 10;
    1 8;
    2 9;
    3 10;
    2 3;
    3 4;
    5 6;
    6 7;
    7 8;
    8 9;
    9 10;
    1 4;
    2 5;
    3 6;
    4 7;
    5 8;
    6 9;
    1 3;
    4 6;
    5 7;
    6 8;
    7 9;
    8 10;
    1 6;
    2 7;
    3 8;
    4 9
    5 10
    4 10
    1 7
    2 8
    4 10];

% G1 LFSR: x^10+x^3+1
s=[0 0 1 0 0 0 0 0 0 1];
n=length(s);
g1=ones(1,n);	%initialization vector for G1

%g=ones(1,38192);
%g2=ones(1,38192);
%gfs=ones(1,38192);

g=ones(1,65536/2);
g2=ones(1,65536/2);
gfs=ones(1,65536/2);

L=2^n-1;

% G2j LFSR: x^10+x^9+x^8+x^6+x^3+x^2+1
t=[0 1 1 0 0 1 0 1 1 1];
q=ones(1,n);	%initialization vector for G2

% generate C/A Code sequences:
tap_sel=tap(sv,:);
for inc=1:L
    g2(:,inc)=mod(sum(q(tap_sel),2),2);
    g(:,inc)=mod(g1(n)+g2(:,inc),2);
   g1=[mod(sum(g1.*s),2) g1(1:n-1)];
   q=[mod(sum(q.*t),2) q(1:n-1)];
end

%upsample to desired rate
if fs~=1
	%fractional upsampling with zero order hold
	index=0;
	for cnt = 1/fs:1/fs:L
		index=index+1;
		if ceil(cnt) > L   %traps a floating point error in index
			gfs(:,index)=g(:,L);
		else
			gfs(:,index)=g(:,ceil(cnt));
		end
	end 
	g=gfs;
end

== matlab function Acquisition_from_autosave/Tracking Loop/Tracking Loops/Tracking Loop3/PRN Generator /MATLAB Function2 ==
  data: u input; I output
function I = fcn(u)

I = cos(u);

== matlab function Acquisition_from_autosave/Tracking Loop/Tracking Loops/Tracking Loop3/PRN Generator /PRN_E ==
  data: array input; y output; shift input
function y = fcn(array, shift)

y = circshift(array, shift);

== matlab function Acquisition_from_autosave/Tracking Loop/Tracking Loops/Tracking Loop2/PRN Generator /MATLAB Function2 ==
  data: u input; I output
function I = fcn(u)

I = cos(u);

== matlab function Acquisition_from_autosave/Tracking Loop/Tracking Loops/Tracking Loop4/Controlled Carrier Generator/MATLAB Function1 ==
  data: f input; wave output; timer input; phase_error input
function wave = NCO(f, timer, phase_error)
wave = exp(1i*(2*pi*f*(timer+phase_error)));

== matlab function Acquisition_from_autosave/Tracking Loop/Tracking Loops/Tracking Loop4/Oscillator/MATLAB Function2 ==
  data: u input; I output; Q output
function [I,Q]= fcn(u)

I = cos(u);
Q = sin(u);

== matlab function Acquisition_from_autosave/Tracking Loop/Tracking Loops/Tracking Loop4/PRN Generator /CA_Code /CA_Code ==
  data: sv input; g output; fs input
function g=CAcode(sv,fs)
coder.extrinsic('warning')
% function G=CACODE(SV,FS) 
% Generates 1023 length C/A Codes for GPS PRNs 1-37
%
% 
% g: nx1023 matrix- with each PRN in each row with symbols 1 and 0
% sv: a row or column vector of the SV's to be generated
% 	 valid entries are 1 to 37
% fs: optional number of samples per chip (defaults to 1), fractional samples allowed, must be 1 or greater.
%
% For multiple samples per chip, function is a zero order hold. 
%
%
% For example to generate the C/A codes for PRN 6 and PRN 12 use:
% g=cacode([6 12]),
% and to generate the C/A codes for PRN 6 and PRN 12 at 5 MHz use
% g=cacode([6 12],5/1.023)
% 
%
% For more information refer to the "GPS SPS Signal Specification"
% http://www.navcen.uscg.gov/pubs/gps/sigspec/default.htm
%
% Dan Boschen 12-30-2007
% boschen@loglin.com

% Revision History
% rev 1.0 Dan Boschen 4-15-2007  Initial Release
%
% rev 1.1 Dan Boschen 7-15-2007  Corrected error with taps for PRN30, should be [2,7] was 
% 					incorrect as [1 7]. Thank you Jadah Zak for finding this.
%
%
% rev 1.2 Dan Boschen 12-26-2007 Fixed column index error when ceil ~ L 
%				Thank you Jared Meadows for finding this.
%
% rev 1.3 Dan Boschen 12-30-2007 Changed comment "first order hold" to
% "zero order hold".
%
% rev 1.4 Dan Boschen 6-1-2010   Updated email address in comments



if nargin<2
	fs=1;
end


if (max(sv)>37) || (min(sv)<1) || (min(size(sv))~=1)
	error('sv must be a row or column vector with integers between 1 and 37\n')
end

if fs<1
	error('fs must be 1 or greater\n')
end	

% force integers
testint=round(sv)-sv;
if testint ~= 0 
	warning('non-integer value entered for sv, rounding to closest integer\n');
	sv = round(sv);
end


% table of C/A Code Tap Selection (sets delay for G2 generator)
tap=[2 6;
    3 7;
    4 8;
    5 9;
    1 9;
    2 10;
    1 8;
    2 9;
    3 10;
    2 3;
    3 4;
    5 6;
    6 7;
    7 8;
    8 9;
    9 10;
    1 4;
    2 5;
    3 6;
    4 7;
    5 8;
    6 9;
    1 3;
    4 6;
    5 7;
    6 8;
    7 9;
    8 10;
    1 6;
    2 7;
    3 8;
    4 9
    5 10
    4 10
    1 7
    2 8
    4 10];

% G1 LFSR: x^10+x^3+1
s=[0 0 1 0 0 0 0 0 0 1];
n=length(s);
g1=ones(1,n);	%initialization vector for G1

%g=ones(1,38192);
%g2=ones(1,38192);
%gfs=ones(1,38192);

g=ones(1,65536/2);
g2=ones(1,65536/2);
gfs=ones(1,65536/2);

L=2^n-1;

% G2j LFSR: x^10+x^9+x^8+x^6+x^3+x^2+1
t=[0 1 1 0 0 1 0 1 1 1];
q=ones(1,n);	%initialization vector for G2

% generate C/A Code sequences:
tap_sel=tap(sv,:);
for inc=1:L
    g2(:,inc)=mod(sum(q(tap_sel),2),2);
    g(:,inc)=mod(g1(n)+g2(:,inc),2);
   g1=[mod(sum(g1.*s),2) g1(1:n-1)];
   q=[mod(sum(q.*t),2) q(1:n-1)];
end

%upsample to desired rate
if fs~=1
	%fractional upsampling with zero order hold
	index=0;
	for cnt = 1/fs:1/fs:L
		index=index+1;
		if ceil(cnt) > L   %traps a floating point error in index
			gfs(:,index)=g(:,L);
		else
			gfs(:,index)=g(:,ceil(cnt));
		end
	end 
	g=gfs;
end

== matlab function Acquisition_from_autosave/Tracking Loop/Tracking Loops/Tracking Loop4/PRN Generator /MATLAB Function2 ==
  data: u input; I output
function I = fcn(u)

I = cos(u);

== matlab function Acquisition_from_autosave/Tracking Loop/Tracking Loops/Tracking Loop2/PRN Generator /PRN_E ==
  data: array input; y output; shift input
function y = fcn(array, shift)

y = circshift(array, shift);

== matlab function Acquisition_from_autosave/Tracking Loop/Tracking Loops/Tracking Loop2/PRN Generator /PRN_L ==
  data: array input; y output; shift input
function y = fcn(array, shift)

y = circshift(array, shift);

== matlab function Acquisition_from_autosave/Tracking Loop/Tracking Loops/Tracking Loop4/PRN Generator /PRN_E ==
  data: array input; y output; shift input
function y = fcn(array, shift)

y = circshift(array, shift);

== matlab function Acquisition_from_autosave/Tracking Loop/MATLAB Function ==
  data: y output
function y = fcn()
%y=[0,1,9207000,0;0,5,9207000,200;0,7,9207000,420;0,9,9207000,999;0,0,0,0;0,0,0,0];
y=[0,1,9207000,0;0,2,9207000,200;0,3,9207000,512;0,4,9207000,999;0,0,0,0;0,0,0,0];

== matlab function Acquisition_from_autosave/Tracking Loop/Tracking Loops/Tracking Loop2/PRN Generator /PRN_P ==
  data: array input; y output size=32768; shift input
function y = fcn(array, shift)

y = circshift(array, shift);

== matlab function Acquisition_from_autosave/Tracking Loop/Tracking Loops/Tracking Loop4/PRN Generator /PRN_L ==
  data: array input; y output; shift input
function y = fcn(array, shift)

y = circshift(array, shift);

== matlab function Acquisition_from_autosave/Tracking Loop/Tracking Loops/Tracking Loop4/PRN Generator /PRN_P ==
  data: array input; y output size=32768; shift input
function y = fcn(array, shift)

y = circshift(array, shift);

== matlab function Acquisition_from_autosave/Tracking Loop/Tracking Loops/Tracking Loop1/Oscillator/MATLAB Function2 ==
  data: u input; I output; Q output
function [I,Q]= fcn(u)

I = cos(u);
Q = sin(u);

== matlab function Acquisition_from_autosave/Tracking Loop/Tracking Loops/Tracking Loop1/PRN Generator /CA_Code /CA_Code ==
  data: sv input; g output; fs input
function g=CAcode(sv,fs)
coder.extrinsic('warning')
% function G=CACODE(SV,FS) 
% Generates 1023 length C/A Codes for GPS PRNs 1-37
%
% 
% g: nx1023 matrix- with each PRN in each row with symbols 1 and 0
% sv: a row or column vector of the SV's to be generated
% 	 valid entries are 1 to 37
% fs: optional number of samples per chip (defaults to 1), fractional samples allowed, must be 1 or greater.
%
% For multiple samples per chip, function is a zero order hold. 
%
%
% For example to generate the C/A codes for PRN 6 and PRN 12 use:
% g=cacode([6 12]),
% and to generate the C/A codes for PRN 6 and PRN 12 at 5 MHz use
% g=cacode([6 12],5/1.023)
% 
%
% For more information refer to the "GPS SPS Signal Specification"
% http://www.navcen.uscg.gov/pubs/gps/sigspec/default.htm
%
% Dan Boschen 12-30-2007
% boschen@loglin.com

% Revision History
% rev 1.0 Dan Boschen 4-15-2007  Initial Release
%
% rev 1.1 Dan Boschen 7-15-2007  Corrected error with taps for PRN30, should be [2,7] was 
% 					incorrect as [1 7]. Thank you Jadah Zak for finding this.
%
%
% rev 1.2 Dan Boschen 12-26-2007 Fixed column index error when ceil ~ L 
%				Thank you Jared Meadows for finding this.
%
% rev 1.3 Dan Boschen 12-30-2007 Changed comment "first order hold" to
% "zero order hold".
%
% rev 1.4 Dan Boschen 6-1-2010   Updated email address in comments



if nargin<2
	fs=1;
end


if (max(sv)>37) || (min(sv)<1) || (min(size(sv))~=1)
	error('sv must be a row or column vector with integers between 1 and 37\n')
end

if fs<1
	error('fs must be 1 or greater\n')
end	

% force integers
testint=round(sv)-sv;
if testint ~= 0 
	warning('non-integer value entered for sv, rounding to closest integer\n');
	sv = round(sv);
end


% table of C/A Code Tap Selection (sets delay for G2 generator)
tap=[2 6;
    3 7;
    4 8;
    5 9;
    1 9;
    2 10;
    1 8;
    2 9;
    3 10;
    2 3;
    3 4;
    5 6;
    6 7;
    7 8;
    8 9;
    9 10;
    1 4;
    2 5;
    3 6;
    4 7;
    5 8;
    6 9;
    1 3;
    4 6;
    5 7;
    6 8;
    7 9;
    8 10;
    1 6;
    2 7;
    3 8;
    4 9
    5 10
    4 10
    1 7
    2 8
    4 10];

% G1 LFSR: x^10+x^3+1
s=[0 0 1 0 0 0 0 0 0 1];
n=length(s);
g1=ones(1,n);	%initialization vector for G1

%g=ones(1,38192);
%g2=ones(1,38192);
%gfs=ones(1,38192);

g=ones(1,65536/2);
g2=ones(1,65536/2);
gfs=ones(1,65536/2);

L=2^n-1;

% G2j LFSR: x^10+x^9+x^8+x^6+x^3+x^2+1
t=[0 1 1 0 0 1 0 1 1 1];
q=ones(1,n);	%initialization vector for G2

% generate C/A Code sequences:
tap_sel=tap(sv,:);
for inc=1:L
    g2(:,inc)=mod(sum(q(tap_sel),2),2);
    g(:,inc)=mod(g1(n)+g2(:,inc),2);
   g1=[mod(sum(g1.*s),2) g1(1:n-1)];
   q=[mod(sum(q.*t),2) q(1:n-1)];
end

%upsample to desired rate
if fs~=1
	%fractional upsampling with zero order hold
	index=0;
	for cnt = 1/fs:1/fs:L
		index=index+1;
		if ceil(cnt) > L   %traps a floating point error in index
			gfs(:,index)=g(:,L);
		else
			gfs(:,index)=g(:,ceil(cnt));
		end
	end 
	g=gfs;
end

== matlab function Acquisition_from_autosave/Tracking Loop/Tracking Loops/Tracking Loop1/PRN Generator /MATLAB Function2 ==
  data: u input; I output
function I = fcn(u)

I = cos(u);

== matlab function Acquisition_from_autosave/Tracking Loop/Tracking Loops/Tracking Loop1/PRN Generator /PRN_E ==
  data: array input; y output; shift input
function y = fcn(array, shift)

y = circshift(array, shift);

== matlab function Acquisition_from_autosave/Tracking Loop/Tracking Loops/Tracking Loop1/PRN Generator /PRN_L ==
  data: array input; y output; shift input
function y = fcn(array, shift)

y = circshift(array, shift);

== matlab function Acquisition_from_autosave/Tracking Loop/Tracking Loops/Tracking Loop3/PRN Generator /PRN_L ==
  data: array input; y output; shift input
function y = fcn(array, shift)

y = circshift(array, shift);

== matlab function Acquisition_from_autosave/Tracking Loop/Tracking Loops/Tracking Loop3/PRN Generator /PRN_P ==
  data: array input; y output size=32768; shift input
function y = fcn(array, shift)

y = circshift(array, shift);

== matlab function Acquisition_from_autosave/Tracking Loop/Tracking Loops/Tracking Loop5/Controlled Carrier Generator/MATLAB Function ==
  data: time input; wave output; freq input; phase input
function wave = NCOGen(time, freq, phase)

wave = exp(1i*(2*pi*freq*time-mod(phase,2*pi)));

== matlab function Acquisition_from_autosave/Tracking Loop/Tracking Loops/Tracking Loop5/Controlled Carrier Generator/MATLAB Function1 ==
  data: f input; wave output; timer input; phase_error input
function wave = NCO(f, timer, phase_error)
wave = exp(1i*(2*pi*f*(timer+phase_error)));
